simulink model "Des_differents_Systemes_De_2eme_Ordre_En_Boucle_Ouverte"  (R2017a)
settings: Solver=VariableStepAuto  StartTime=0.0  StopTime=100  RelTol=1e-3
values from neighbouring files (symbols this model uses):
  K1 = 1    [declarationDesVariables.m]
  K2 = 5    [declarationDesVariables.m]
  K3 = 10    [declarationDesVariables.m]
  L1 = 0.2    [declarationDesVariables.m]
  L2 = 0.7    [declarationDesVariables.m]
  L3 = 1    [declarationDesVariables.m]
  Wn1 = 1    [declarationDesVariables.m]
  Wn2 = 2    [declarationDesVariables.m]
  Wn3 = 5    [declarationDesVariables.m]
settings Model: Creator=PC  LastModifiedBy=PC

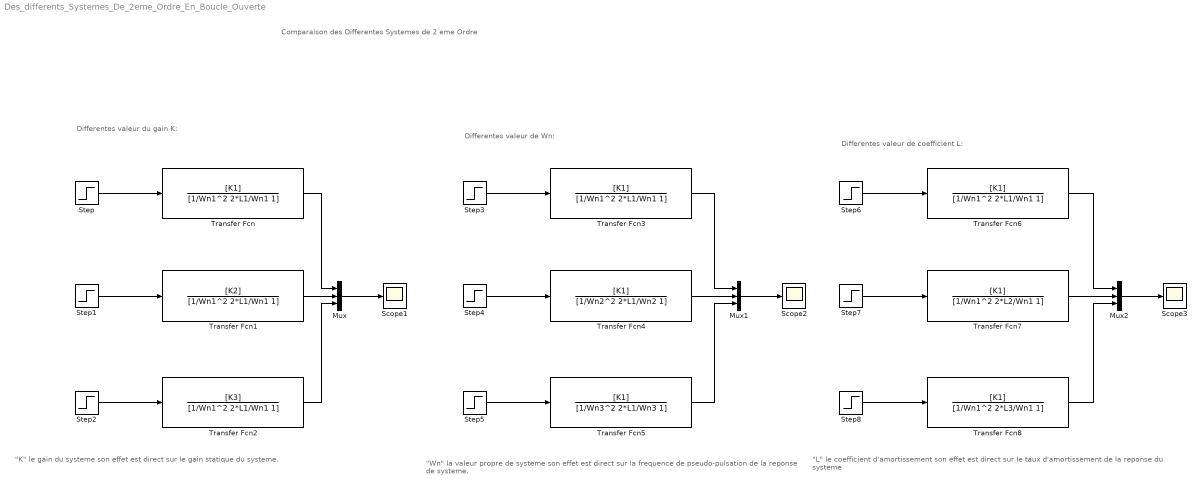
== system Des_differents_Systemes_De_2eme_Ordre_En_Boucle_Ouverte ==
  note: Differentes valeur du gain K:
  note: "L" le coefficient d'amortissement
      | son effet est direct sur le taux d'amortissement de
      | la reponse du systeme
  note: Comparaison des Differentes Systemes de 2 eme Ordre
  note: "Wn" la valeur propre de systeme son effet est direct sur la frequence de pseudo-pulsation de la reponse de systeme.
  note: "K" le gain du systeme son effet est direct sur le gain statique
      | du systeme.
  note: Differentes valeur de Wn:
  note: Differentes valeur de coefficient L:
  Mux : Mux  Inputs=3
  Mux1 : Mux  Inputs=3
  Mux2 : Mux  Inputs=3
  Scope1 : Scope
  Scope2 : Scope
  Scope3 : Scope
  Step{,1..8} (9 alike) : Step  SampleTime=0
  Transfer Fcn : TransferFcn  Numerator=[K1]  Denominator=[1/Wn1^2 2*L1/Wn1 1]
  Transfer Fcn1 : TransferFcn  Numerator=[K2]  Denominator=[1/Wn1^2 2*L1/Wn1 1]
  Transfer Fcn2 : TransferFcn  Numerator=[K3]  Denominator=[1/Wn1^2 2*L1/Wn1 1]
  Transfer Fcn3 : TransferFcn  Numerator=[K1]  Denominator=[1/Wn1^2 2*L1/Wn1 1]
  Transfer Fcn4 : TransferFcn  Numerator=[K1]  Denominator=[1/Wn2^2 2*L1/Wn2 1]
  Transfer Fcn5 : TransferFcn  Numerator=[K1]  Denominator=[1/Wn3^2 2*L1/Wn3 1]
  Transfer Fcn6 : TransferFcn  Numerator=[K1]  Denominator=[1/Wn1^2 2*L1/Wn1 1]
  Transfer Fcn7 : TransferFcn  Numerator=[K1]  Denominator=[1/Wn1^2 2*L2/Wn1 1]
  Transfer Fcn8 : TransferFcn  Numerator=[K1]  Denominator=[1/Wn1^2 2*L3/Wn1 1]
  wires:
  Step/1 -> Transfer Fcn/1
  Step1/1 -> Transfer Fcn1/1
  Step2/1 -> Transfer Fcn2/1
  Step5/1 -> Transfer Fcn5/1
  Step4/1 -> Transfer Fcn4/1
  Step3/1 -> Transfer Fcn3/1
  Step6/1 -> Transfer Fcn6/1
  Step7/1 -> Transfer Fcn7/1
  Step8/1 -> Transfer Fcn8/1
  Mux/1 -> Scope1/1
  Transfer Fcn/1 -> Mux/1
  Transfer Fcn1/1 -> Mux/2
  Transfer Fcn2/1 -> Mux/3
  Mux1/1 -> Scope2/1
  Transfer Fcn4/1 -> Mux1/2
  Transfer Fcn3/1 -> Mux1/1
  Transfer Fcn5/1 -> Mux1/3
  Transfer Fcn6/1 -> Mux2/1
  Mux2/1 -> Scope3/1
  Transfer Fcn7/1 -> Mux2/2
  Transfer Fcn8/1 -> Mux2/3
